simulink model "successive_over_relaxation"  (R2021a)
settings: Solver=FixedStepDiscrete  StartTime=0.0  StopTime=10  FixedStep=1  RelTol=1e-3
libraries: dspmtrx3 x4, dspinverses x1, simulink x1
settings Model: Creator=manur  LastModifiedBy=manur

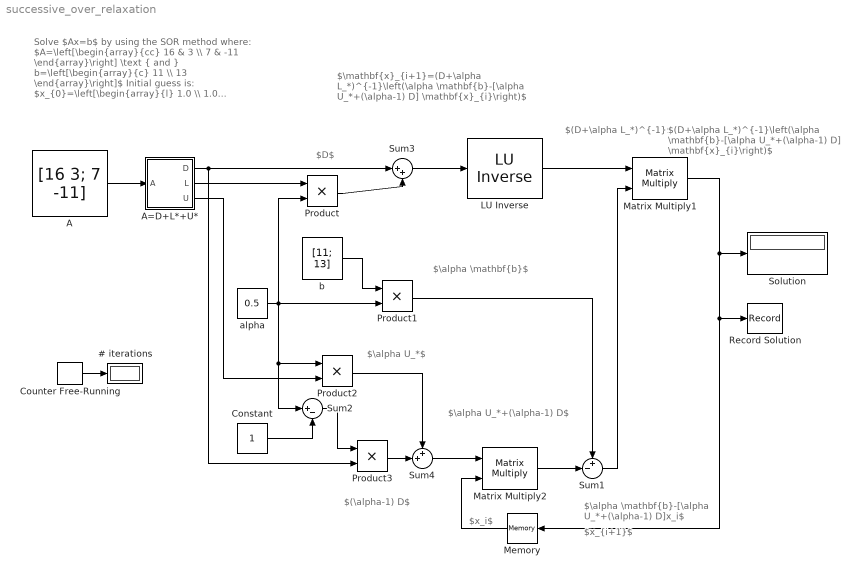
== system successive_over_relaxation ==
  note: $\alpha \mathbf{b}-[\alpha U_*+(\alpha-1) D]x_i$
  note: $\alpha \mathbf{b}$
  note: $\mathbf{x}_{i+1}=(D+\alpha L_*)^{-1}\left(\alpha \mathbf{b}-[\alpha U_*+(\alpha-1) D] \mathbf{x}_{i}\right)$
  note: Solve $Ax=b$ by using the SOR method where:
      | $A=\left[\begin{array}{cc} 16 & 3 \\ 7 & -11 \end{array}\right] \text { and } b=\left[\begin{array}{c} 11 \\ 13 \end{array}\right]$
      | Initial guess is:
      | $x_{0}=\left[\begin{array}{l} 1.0 \\ 1.0 \end{array}\right]$
      | Set $\alpha=0.5$
  note: $D$
  note: $(D+\alpha L_*)^{-1}$
  note: $x_i$
  note: $x_{i+1}$
  note: $\alpha U_*$
  note: $(\alpha-1) D$
  note: $\alpha U_*+(\alpha-1) D$
  note: $(D+\alpha L_*)^{-1}\left(\alpha \mathbf{b}-[\alpha U_*+(\alpha-1) D] \mathbf{x}_{i}\right)$
  " LU Inverse" : dspinverses/ LU Inverse
  # iterations : Display
  A : Constant  Value=[16 3; 7 -11]
  A=D+L*+U* : Subsystem
      mask Display: image('$imagefile'); % Use "Edit Image" on toolstrip to change.
  Constant : Constant
  Counter Free-Running : simulink/Sources/Counter Free-Running  NumBits=16  tsamp=-1
  Matrix Multiply1 : Product  Multiplication=Matrix(*)
  Matrix Multiply2 : Product  Multiplication=Matrix(*)
  Memory : Memory  InitialCondition=[1; 1]
  Product{,1..3} (4 alike) : Product
  Record Solution : Record  FileSettingsInternal="{\"entries\":[{\"content\":{\"excelSettings\":{\"content\":{},\"type\":\"Streamout.ExcelSettings\"}},\"type\":\"Streamout.FileSettingStorage\",\"uuid\":\"443e61f6-5447-4ec9-a7f4-f5e5c8be4017\"}],\"packageUris\":[\"http://schema.mathworks.com/mf0/streamout_blocks/R2020a\"],\"version\":\"1.0\"}"  Layout=[1 1]  SignalsInternal="{\"entries\":[{\"content\":{\"signals\":[{\"content\":{\"blockPath\":[\"xuccessive_over_relaxation/Record Solution\"],\"channel\":[],\"dimensions\":[2,1],\"domain\":\"xuccessive_over_relaxation/record solution\",\"hasChildren\":true,\"lineColor\":\"#0072bd\",\"plots\":[],\"port\":1,\"sid\":[\"\"],\"signalID\":303,\"signalName\":\"Matrix Multiply1\"},\"type\":\"RecordBlkView.Signal\",\"uuid\":\"02c71bc3-add5-43f9-ba33-aa2eabd385ab\"},{\"content\":{\"blockPath\":[\"xuccessive_over_relaxation/Record Solution\"],\"channel\":[1,1],\"dimensions\":[2,1],\"domain\":\"xuccessive_over_relaxation/record solution\",\"lineColor\":\"#7e2f8e\",\"parentID\":303,\"plots\":[1],\"port\":1,\"sid\":[\"\"],\"signalID\":304,\"signalName\":\"Matrix Multiply1\"},\"type\":\"RecordBlkView.Signal\",\"uuid\":\"924404e6-a3af-42ff-aa42-135474c67496\"}]},\"type\":\"RecordBlkView.InputSignals\",\"uuid\":\"a8d933ee-060e-4344-96ef-520bd3125ef3\"}],\"packageUris\":[\"http://schema.mathworks.com/mf0/streamout_blocks/R2020a\"],\"version\":\"1.0\"}"  VisualizationBindings="{\"sparklinesplugin\":{\"info\":[{\"bindingParametersList\":[],\"subplotID\":1}]}}"
  Solution : Display
  Sum1 : Sum  Inputs=+-|
  Sum2 : Sum  Inputs=|+-
  Sum3 : Sum  Inputs=|++
  Sum4 : Sum  Inputs=++|
  alpha : Constant  Value=0.5
  b : Constant  Value=[11; 13]  VectorParams1D=off
  wires:
  Counter Free-Running/1 -> # iterations/1
  A/1 -> A=D+L*+U*/1(A)
  " LU Inverse"/1 -> Matrix Multiply1/1
  Matrix Multiply1/1 -> Record Solution/1, Memory/1, Solution/1
  Memory/1 -> Matrix Multiply2/2
  b/1 -> Product1/1
  A=D+L*+U*/1(D) -> Product3/2, Sum3/1
  A=D+L*+U*/2(L) -> Product/1
  A=D+L*+U*/3(U) -> Product2/2
  Sum3/1 -> " LU Inverse"/1
  Product/1 -> Sum3/2
  Product3/1 -> Sum4/2
  Product2/1 -> Sum4/1
  Sum4/1 -> Matrix Multiply2/1
  Matrix Multiply2/1 -> Sum1/2
  Product1/1 -> Sum1/1
  Sum1/1 -> Matrix Multiply1/2
  alpha/1 -> Sum2/1, Product2/1, Product/2, Product1/2
  Sum2/1 -> Product3/1
  Constant/1 -> Sum2/2

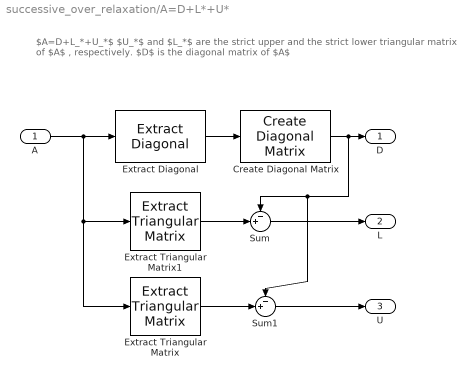
== system successive_over_relaxation/A=D+L*+U* ==
  note: $A=D+L_*+U_*$
      | $U_*$ and $L_*$ are the strict upper and the strict lower triangular matrix of $A$ , respectively.
      | $D$ is the diagonal matrix of $A$
  A : Inport
  Create Diagonal Matrix : dspmtrx3/Create Diagonal Matrix
      settings: SourceProductBaseCode=DS
  Extract Diagonal : dspmtrx3/Extract Diagonal
      settings: SourceProductBaseCode=DS
  Extract Triangular Matrix : dspmtrx3/Extract Triangular Matrix  fcn=Upper  SimulateUsing=Code generation
      settings: SourceProductBaseCode=DS
  Extract Triangular Matrix1 : dspmtrx3/Extract Triangular Matrix  fcn=Lower  SimulateUsing=Code generation
      settings: SourceProductBaseCode=DS
  Sum : Sum  Inputs=-+|
  Sum1 : Sum  Inputs=-+|
  D : Outport
  L : Outport  Port=2
  U : Outport  Port=3
  wires:
  Extract Diagonal/1 -> Create Diagonal Matrix/1
  A/1 -> Extract Diagonal/1, Extract Triangular Matrix1/1, Extract Triangular Matrix/1
  Create Diagonal Matrix/1 -> D/1, Sum1/1, Sum/1
  Sum/1 -> L/1
  Extract Triangular Matrix1/1 -> Sum/2
  Extract Triangular Matrix/1 -> Sum1/2
  Sum1/1 -> U/1
